simulink model "RI_ISZM"  (R2013b)
settings: Solver=ode45  StartTime=0.0  StopTime=1e-3  RelTol=1e-3
libraries: RI_MK x2
settings Model: Creator=Szalay  LastModifiedBy=Szalay

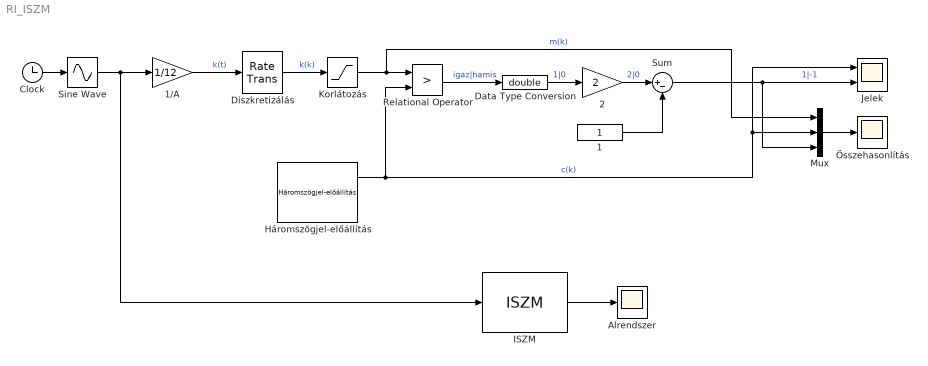
== system RI_ISZM ==
  1 : Constant
  1/A : Gain  Gain=1/12
  2 : Gain  Gain=2
  Alrendszer : Scope
      settings: ShowLegends=on  SaveName=ScopeData2
  Clock : Clock
  Data Type Conversion : DataTypeConversion  OutDataTypeStr=double
  Diszkretizálás : RateTransition  OutPortSampleTime=50e-6
  Háromszögjel-előállítás : RI_MK/Háromszögjel-előállítás  T_S=1e-6  A=1  f=10000
  ISZM : RI_MK/ISZM  U_T=12  f_ISZM=10000  T_S=1e-6
  Jelek : Scope  NumInputPorts=2
      settings: ShowLegends=on  TimeRange=0.0006000000000000001  YMin=-15~-1  YMax=15~2
  Korlátozás : Saturate  UpperLimit=12-0.5  LowerLimit=-12+0.5
  Mux : Mux  Inputs=3
  Relational Operator : RelationalOperator  Operator=>  OutDataTypeStr=boolean
  Sine Wave : Sin  TimeSource=Use external signal  Amplitude=12  Frequency=2*pi*(1/1000e-6)  SampleTime=0
  Sum : Sum  Inputs=|+-
  Összehasonlítás : Scope
      settings: TimeRange=0.001  YMin=-1.5  YMax=1.5
  wires:
  Háromszögjel-előállítás/1 -> Relational Operator/2, Mux/2, Jelek/1  "c(k)"
  Sine Wave/1 -> ISZM/1, 1/A/1
  Relational Operator/1 -> Data Type Conversion/1  "igaz|hamis"
  Mux/1 -> Összehasonlítás/1
  Sum/1 -> Jelek/2, Mux/3  "1|-1"
  Clock/1 -> Sine Wave/1
  Diszkretizálás/1 -> Korlátozás/1  "k(k)"
  Korlátozás/1 -> Relational Operator/1, Mux/1  "m(k)"
  1/A/1 -> Diszkretizálás/1  "k(t)"
  Data Type Conversion/1 -> 2/1  "1|0"
  2/1 -> Sum/1  "2|0"
  1/1 -> Sum/2
  ISZM/1 -> Alrendszer/1
